simulink model "small_signal_verification"  (R2021a)
settings: Solver=VariableStepAuto  StartTime=0.0  StopTime=t_sim  RelTol=1e-3
values from neighbouring files (symbols this model uses):
  C = 600e-6    (= 0.0006)    [boost_parameters.m]    (also in buck_parameters.m = 0.0002)
  D = (Vref-Vin)/Vref    (= 0.5)    [boost_parameters.m]    (also in buck_parameters.m = 0.1; small_signal_model.m = 0.1)
  delta_Io = 0    [small_signal_model.m]
  delta_Vcon = delta_D*V_m    (= 0)    [small_signal_model.m]
  delta_Vin = -2    [small_signal_model.m]
  iL_0 = 0    [boost_parameters.m]    (also in buck_parameters.m)
  L = 50e-6    (= 5e-05)    [boost_parameters.m]    (also in buck_parameters.m = 5e-07)
  R = 1    [boost_parameters.m]    (also in buck_parameters.m; small_signal_model.m = 10; soft_start.m; soft_start_feedforward_backward.m)
  r_1 = 5e-3    (= 0.005)    [boost_parameters.m]    (also in buck_parameters.m)
  r_2 = 5e-3    (= 0.005)    [boost_parameters.m]    (also in buck_parameters.m)
  r_C = 3e-3    (= 0.003)    [boost_parameters.m]    (also in buck_parameters.m)
  r_L = 5e-3    (= 0.005)    [boost_parameters.m]    (also in buck_parameters.m)
  T = 2e-6    (= 2e-06)    [boost_parameters.m]    (also in buck_parameters.m)
  t_step = 2e-3    (= 0.002)    [small_signal_model.m]
  V_m = 10    [small_signal_model.m]    (also in soft_start.m; soft_start_feedforward_backward.m; without_soft_start.m)
  vC_0 = 0    [boost_parameters.m]    (also in buck_parameters.m)
  Vcon = D*V_m    (= 1)    [small_signal_model.m]
  Vin = 12    [boost_parameters.m]    (also in buck_parameters.m; small_signal_model.m)
libraries: simulink x1, simulink_extras x1
settings Model: Creator=Hari Prasad Adhikari  LastModifiedBy=Hari Prasad Adhikari

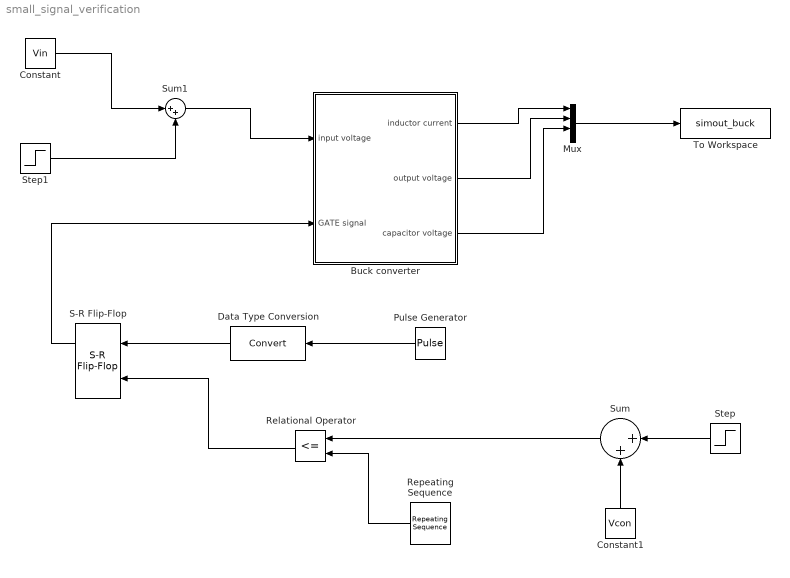
== system small_signal_verification ==
  Buck converter : Subsystem
  Constant : Constant  Value=Vin
  Constant1 : Constant  Value=Vcon
  Data Type Conversion : DataTypeConversion  OutMin=[0]  OutMax=[1]
  Mux : Mux
  Pulse Generator : DiscretePulseGenerator  PulseType=Time based  Period=T  PulseWidth=D*100
  Relational Operator : RelationalOperator  Operator=<=  OutDataTypeStr=boolean  RndMeth=Simplest
  Repeating Sequence : simulink/Sources/Repeating Sequence  rep_seq_t=[0 T]  rep_seq_y="[0  V_m]"
  S-R Flip-Flop : simulink_extras/Flip Flops/S-R Flip-Flop  initial_condition=0
  Step : Step  Time=t_step  After=delta_Vcon  SampleTime=0
  Step1 : Step  Time=t_step  After=delta_Vin  SampleTime=0
  Sum : Sum  Inputs=|++
  Sum1 : Sum  Inputs=|++
  To Workspace : ToWorkspace  VariableName=simout_buck  SaveFormat=Timeseries  SampleTime=-1
  wires:
  Buck converter/1(inductor current) -> Mux/1
  Buck converter/2(output voltage) -> Mux/2
  Buck converter/3(capacitor voltage) -> Mux/3
  Mux/1 -> To Workspace/1
  S-R Flip-Flop/1 -> Buck converter/2(GATE signal)
  Constant1/1 -> Sum/2
  Step/1 -> Sum/1
  Pulse Generator/1 -> Data Type Conversion/1
  Data Type Conversion/1 -> S-R Flip-Flop/1
  Sum/1 -> Relational Operator/1
  Repeating Sequence/1 -> Relational Operator/2
  Relational Operator/1 -> S-R Flip-Flop/2
  Constant/1 -> Sum1/1
  Sum1/1 -> Buck converter/1(input voltage)
  Step1/1 -> Sum1/2

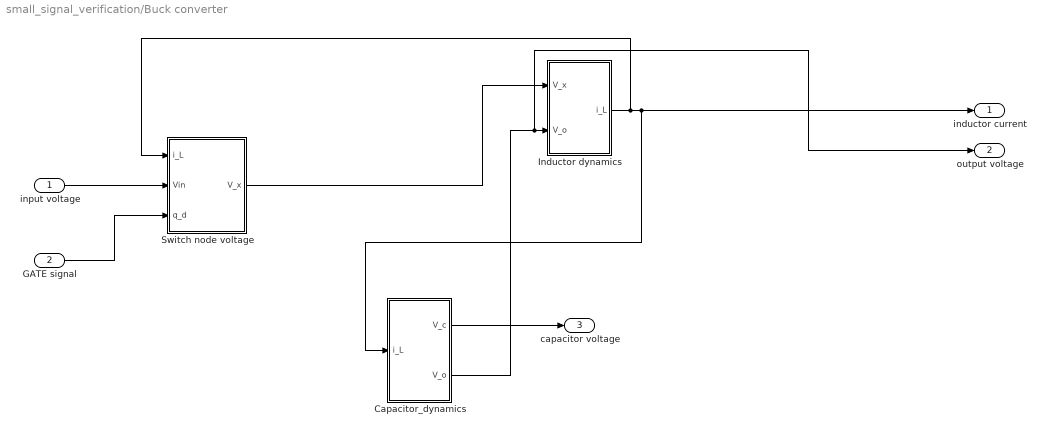
== system small_signal_verification/Buck converter ==
  input voltage : Inport
  GATE signal : Inport  Port=2
  Capacitor_dynamics : Subsystem
  Inductor dynamics : Subsystem
  Switch node voltage : Subsystem
  inductor current : Outport
  output voltage : Outport  Port=2
  capacitor voltage : Outport  Port=3
  wires:
  Capacitor_dynamics/1(V_c) -> capacitor voltage/1
  Inductor dynamics/1(i_L) -> inductor current/1, Capacitor_dynamics/1(i_L), Switch node voltage/1(i_L)
  Capacitor_dynamics/2(V_o) -> output voltage/1, Inductor dynamics/2(V_o)
  Switch node voltage/1(V_x) -> Inductor dynamics/1(V_x)
  GATE signal/1 -> Switch node voltage/3(q_d)
  input voltage/1 -> Switch node voltage/2(Vin)

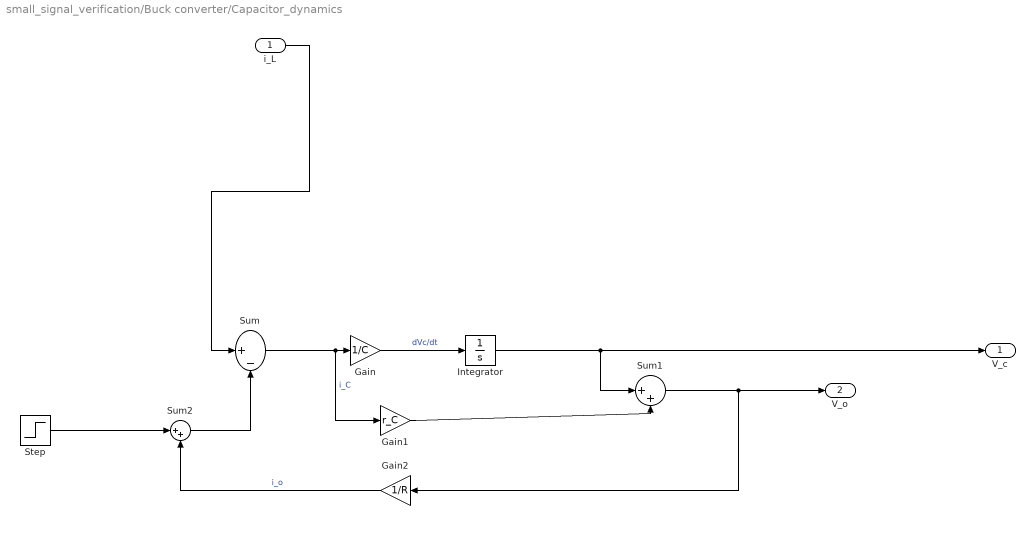
== system small_signal_verification/Buck converter/Capacitor_dynamics ==
  i_L : Inport
  Gain : Gain  Gain=1/C
  Gain1 : Gain  Gain=r_C
  Gain2 : Gain  Gain=1/R
  Integrator : Integrator  InitialCondition=vC_0
  Step : Step  Time=t_step  After=delta_Io  SampleTime=0
  Sum : Sum  Inputs=|+-
  Sum1 : Sum  Inputs=|++
  Sum2 : Sum  Inputs=|++
  V_c : Outport
  V_o : Outport  Port=2
  wires:
  Integrator/1 -> V_c/1, Sum1/1
  Sum1/1 -> V_o/1, Gain2/1
  Gain1/1 -> Sum1/2
  Sum/1 -> Gain1/1, Gain/1  "i_C"
  Gain/1 -> Integrator/1  "dVc/dt"
  i_L/1 -> Sum/1
  Step/1 -> Sum2/1
  Gain2/1 -> Sum2/2  "i_o"
  Sum2/1 -> Sum/2

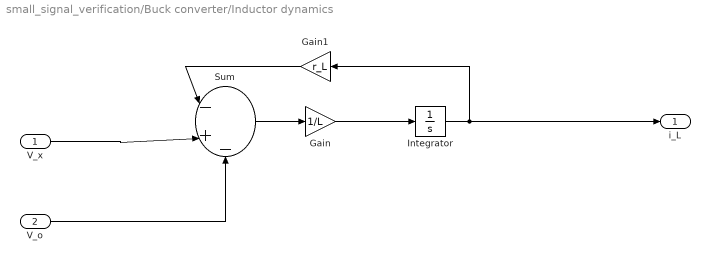
== system small_signal_verification/Buck converter/Inductor dynamics ==
  V_x : Inport
  V_o : Inport  Port=2
  Gain : Gain  Gain=1/L
  Gain1 : Gain  Gain=r_L
  Integrator : Integrator  InitialCondition=iL_0
  Sum : Sum  Inputs=|-+-
  i_L : Outport
  wires:
  Integrator/1 -> i_L/1, Gain1/1
  Gain/1 -> Integrator/1
  V_o/1 -> Sum/3
  Sum/1 -> Gain/1
  Gain1/1 -> Sum/1
  V_x/1 -> Sum/2

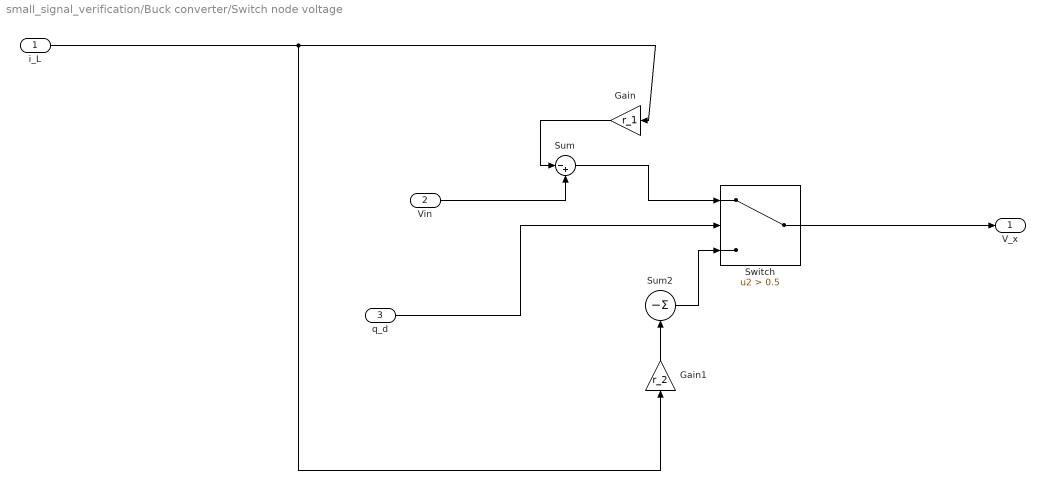
== system small_signal_verification/Buck converter/Switch node voltage ==
  i_L : Inport
  Vin : Inport  Port=2
  q_d : Inport  Port=3
  Gain : Gain  Gain=r_1
  Gain1 : Gain  Gain=r_2
  Sum : Sum  Inputs=|-+
  Sum2 : Sum  Inputs=|-
  Switch : Switch  Criteria=u2 > Threshold  Threshold=0.5
  V_x : Outport
  wires:
  Gain/1 -> Sum/1
  Gain1/1 -> Sum2/1
  i_L/1 -> Gain1/1, Gain/1
  Switch/1 -> V_x/1
  Sum/1 -> Switch/1
  q_d/1 -> Switch/2
  Sum2/1 -> Switch/3
  Vin/1 -> Sum/2
